simulink model "experimental_results"  (R2020b)
settings: Solver=ode1  StartTime=0.0  StopTime=60  FixedStep=0.002  RelTol=1e-3  EnableMultiTasking=on
PreLoadFcn:
  | quanser_aero_lqr
undefined symbols (not defined in the file or in its folder): HIL, qc_get_step_size
libraries: quarc_library x6
settings Model: SimulationMode=external  ExtModeTrigDuration=20000  Creator=MLevis  LastModifiedBy=ffsandva
settings SolverCC: PositivePriorityOrder=on
settings DataIOCC: LimitDataPoints=on  SaveFormat=Array  ReturnWorkspaceOutputs=off
settings OptimizationCC: LifeSpan=inf
settings DebuggingCC: SolverPrmCheckMsg=warning  SFUnexpectedBacktrackingDiag=warning  SFNoUnconditionalDefaultTransitionDiag=warning  SFExecutionAtInitializationDiag=none  ArithmeticOperatorsInVariantConditions=warning
settings HardwareCC: ProdBitPerPointer=32  ProdBitPerSizeT=32  ProdBitPerPtrDiffT=32  ProdLargestAtomicFloat=None  ProdIntDivRoundTo=Undefined  ProdEndianess=Unspecified  ProdWordSize=32  ProdHWDeviceType=32-bit Generic
settings ModelReferenceCC: PropagateSignalLabelsOutOfModel=off
settings SFSimCC: SimUseLocalCustomCode=off  CustomCodeUndefinedFunction=UseInterfaceOnly
settings RTWCC: Description=QUARC Win64 Target  SystemTargetFile=quarc_win64.tlc  TemplateMakefile=quarc_default_tmf  RTWUseLocalCustomCode=off
settings CodeAppCC: StateflowObjectComments=on
settings STFCustomTargetCC: CPPClassGenCompliant=off
settings GRTTargetCC: TargetLangStandard=C89/C90 (ANSI)  ParMdlRefBuildCompliant=off  CompOptLevelCompliant=off  CombineOutputUpdateFcns=off  MatFileLogging=off  CPPClassGenCompliant=off  GRTInterface=on  UseToolchainInfoCompliant=off  ExtMode=on  ExtModeMexFile=quarc_comm
settings ConfigComp: CovMetricSettings=dw  CovSaveCumulativeToWorkspaceVar=on  CovSaveSingleToWorkspaceVar=on  CovExternalEMLEnable=off  CovSFcnEnable=off

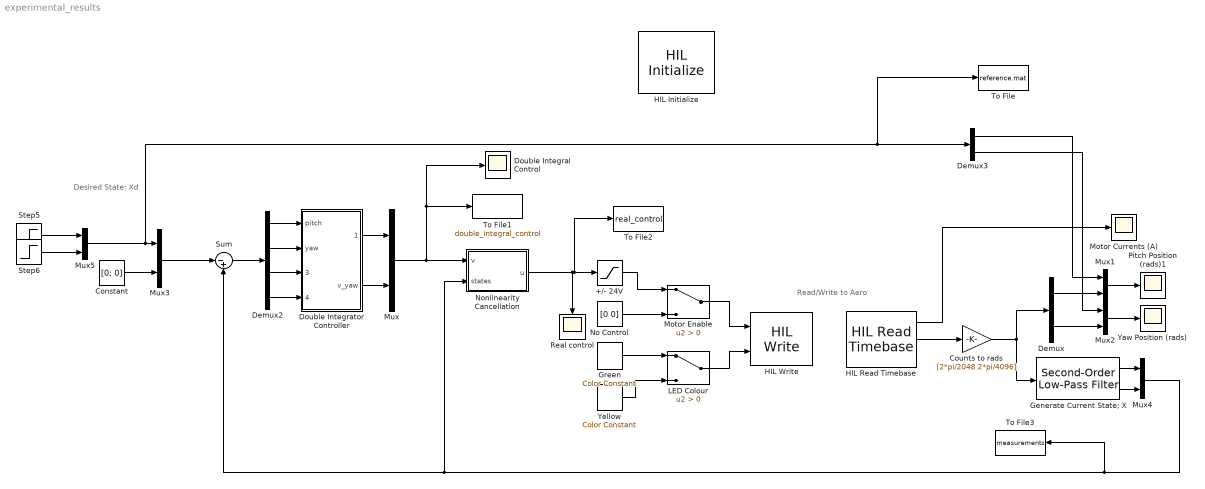
== system experimental_results ==
  note: Read/Write to Aero
  note: Desired State; Xd
  +/- 24V : Saturate  UpperLimit=24  LowerLimit=-24
  Constant : Constant  Value=[0; 0]
  Counts to rads : Gain  Gain=[2*pi/2048 2*pi/4096]
  Demux : Demux  Outputs=2
  Demux2 : Demux
  Demux3 : Demux  Outputs=2
  Double Integral Control : Scope
  Double Integrator Controller : Subsystem
  Generate Current State; X : quarc_library/Continuous/Second-Order Low-Pass Filter  params_source=Internal (dialog parameters)  input_width=50  input_zeta=0.8  input_init=0
  Green : quarc_library/Sources/Signals/Color Constant  color=[0 1 0]
      settings: SourceProductName=QUARC Targets
  HIL Initialize : quarc_library/Data Acquisition/Generic/Configuration/HIL Initialize  Priority=-99  object_name=HIL-1  board_type=quanser_aero_usb  board_number=0  board_options=""  exclusive=off  active=off  hardware_clocks=[0]  clock_modes=[]  initial_clock_frequencies=[]  set_clock_params_at_start=off  set_clock_params_at_switch_in=off  set_clock_frequencies_at_start=off  set_clock_frequencies_at_switch_in=off  analog_input_channels=[0:1]  analog_input_configurations=[]  analog_input_maximums=3  analog_input_minimums=-3  set_analog_input_params_at_start=off  set_analog_input_params_at_switch_in=off  analog_output_channels=[0:1]  analog_output_maximums=24  analog_output_minimums=-24  initial_analog_outputs=[0]  final_analog_outputs=[0]  watchdog_analog_outputs=[0]  set_analog_output_params_at_start=off  set_analog_output_params_at_switch_in=off  set_analog_outputs_at_start=on  set_analog_outputs_at_switch_in=off  set_analog_outputs_at_terminate=on  set_analog_outputs_at_switch_out=off  set_analog_outputs_on_watchdog=on  digital_input_channels=[]  digital_output_channels=[0:1]  digital_output_configuration=[]  initial_digital_outputs=[1]  final_digital_outputs=[0]  watchdog_digital_outputs=[0]  set_digital_output_params_at_start=off  set_digital_output_params_at_switch_in=off  set_digital_outputs_at_start=on  set_digital_outputs_at_switch_in=off  set_digital_outputs_at_terminate=on  set_digital_outputs_at_switch_out=off  set_digital_outputs_on_watchdog=on  encoder_channels=[0:3]  quadrature=[4]  encoder_filter_frequency=[]  initial_encoder_counts=[0]  set_encoder_params_at_start=off  set_encoder_params_at_switch_in=off  set_encoder_counts_at_start=on  set_encoder_counts_at_switch_in=off  pwm_channels=[]  pwm_modes=[]  pwm_frequency=[]  pwm_configuration=[]  pwm_alignment=[]  pwm_polarity=[]  pwm_leading_deadband=[]  pwm_trailing_deadband=[]  initial_pwm_outputs=[]  final_pwm_outputs=[]  watchdog_pwm_outputs=[]  set_pwm_params_at_start=off  set_pwm_params_at_switch_in=off  set_pwm_outputs_at_start=off  set_pwm_outputs_at_switch_in=off  set_pwm_outputs_at_terminate=off  set_pwm_outputs_at_switch_out=off  set_pwm_outputs_on_watchdog=off  other_output_channels=[11000:11002]  initial_other_outputs=[0 1 0]  final_other_outputs=[1 0 0]  watchdog_other_outputs=[0 0 1]  set_other_outputs_at_start=on  set_other_outputs_at_switch_in=off  set_other_outputs_at_terminate=on  set_other_outputs_at_switch_out=off  set_other_outputs_on_watchdog=on
  HIL Read Timebase : quarc_library/Data Acquisition/Generic/Timebases/HIL Read Timebase  object_name=HIL-1  clock=0  analog_channels=[0:1]  encoder_channels=[2:3]  digital_channels=[]  other_channels=[4000 4002 14000 14001]  active=on  vector_output=on  data_type_mode=Inherit via back propagation  encoder_data_type=double  digital_data_type=boolean  overflow_mode=Error on overflow  samples_in_buffer=max(ceil(1/qc_get_step_size), 1)
  HIL Write : quarc_library/Data Acquisition/Generic/Immediate I//O/HIL Write  object_name=HIL-1  analog_channels=[0:1]  pwm_channels=[]  digital_channels=[]  other_channels=[11000:11002]  sample_time=-1  active=off  vector_input=on
  LED Colour : Switch  Criteria=u2 > Threshold
  Motor Currents (A) : Scope
  Motor Enable : Switch  Criteria=u2 > Threshold
  Mux{,1..5} (6 alike) : Mux  Inputs=2
  No Control : Constant  Value=[0 0]
  Nonlinearity Cancellation : MATLAB Function  TreatAsAtomicUnit=on
  Pitch Position (rads)1 : Scope
  Real control : Scope
  Step5 : Step  Time=5  After=pi/6  SampleTime=0
  Step6 : Step  Time=5  After=pi/4  SampleTime=0
  Sum : Sum  Inputs=|-+
  To File : ToFile  Filename=reference.mat
  To File1 : ToFile  Filename=double_integral_control
  To File2 : ToFile  Filename=real_control
  To File3 : ToFile  Filename=measurements
  Yaw Position (rads) : Scope
  Yellow : quarc_library/Sources/Signals/Color Constant  color=[1 1 0]
      settings: SourceProductName=QUARC Targets
  wires:
  HIL Read Timebase/2 -> Counts to rads/1
  +/- 24V/1 -> Motor Enable/1
  Motor Enable/1 -> HIL Write/1
  LED Colour/1 -> HIL Write/2
  No Control/1 -> Motor Enable/3
  Green/1 -> LED Colour/1
  Yellow/1 -> LED Colour/3
  Counts to rads/1 -> Demux/1, Generate Current State; X/1
  HIL Read Timebase/1 -> Motor Currents (A)/1
  Generate Current State; X/2 -> Mux4/2
  Generate Current State; X/1 -> Mux4/1
  Demux/1 -> Mux1/2
  Mux1/1 -> Pitch Position (rads)1/1
  Demux/2 -> Mux2/2
  Mux2/1 -> Yaw Position (rads)/1
  Mux4/1 -> To File3/1, Sum/2, Nonlinearity Cancellation/2(states)
  Double Integrator Controller/1(v_pitch) -> Mux/1
  Double Integrator Controller/2(v_yaw) -> Mux/2
  Demux2/1 -> Double Integrator Controller/1(pitch)
  Demux2/2 -> Double Integrator Controller/2(yaw)
  Demux2/3 -> Double Integrator Controller/3(pitch_dot)
  Demux2/4 -> Double Integrator Controller/4(yaw_dot)
  Sum/1 -> Demux2/1
  Mux5/1 -> To File/1, Demux3/1, Mux3/1
  Constant/1 -> Mux3/2
  Mux3/1 -> Sum/1
  Demux3/1 -> Mux1/1
  Demux3/2 -> Mux2/1
  Mux/1 -> Double Integral Control/1, To File1/1, Nonlinearity Cancellation/1(v)
  Nonlinearity Cancellation/1(u) -> Real control/1, To File2/1, +/- 24V/1
  Step6/1 -> Mux5/2
  Step5/1 -> Mux5/1

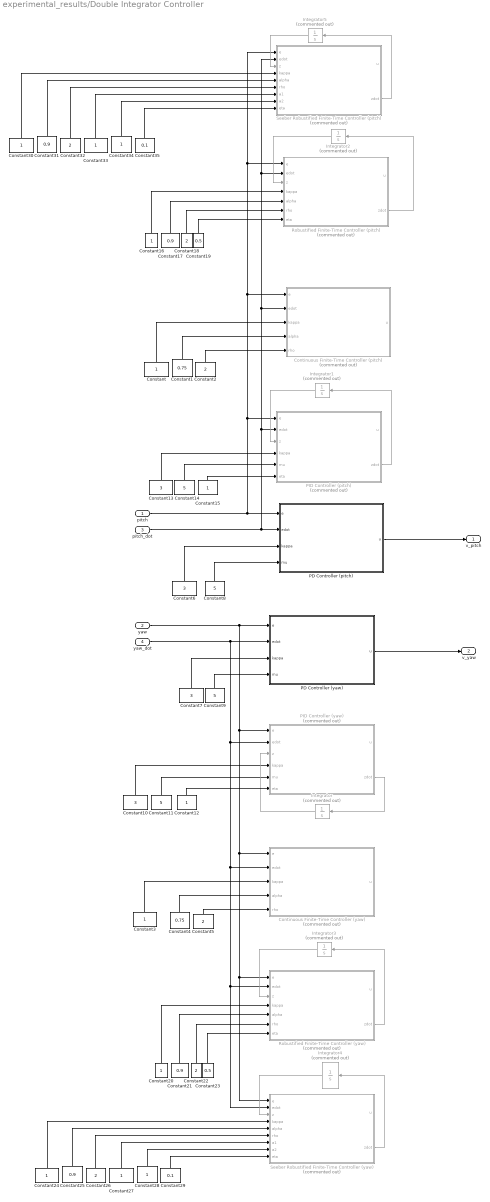
== system experimental_results/Double Integrator Controller ==
  pitch : Inport
  yaw : Inport  Port=2
  pitch_dot : Inport  Port=3
  yaw_dot : Inport  Port=4
  Constant{,3,12,15..16,20,24,27..28,30,33..34} (12 alike) : Constant
  Constant1 : Constant  Value=0.75
  Constant{6..7,10,13} (4 alike) : Constant  Value=3
  Constant{8..9,11,14} (4 alike) : Constant  Value=5
  Constant{17,21,25,31} (4 alike) : Constant  Value=0.9
  Constant{2,5,18,22,26,32} (6 alike) : Constant  Value=2
  Constant19 : Constant  Value=0.5
  Constant23 : Constant  Value=0.5
  Constant29 : Constant  Value=0.1
  Constant35 : Constant  Value=0.1
  Constant4 : Constant  Value=0.75
  Continuous Finite-Time Controller (pitch) : MATLAB Function  Commented=on  TreatAsAtomicUnit=on
  Continuous Finite-Time Controller (yaw) : MATLAB Function  Commented=on  TreatAsAtomicUnit=on
  Integrator{,1..5} (6 alike) : Integrator  Commented=on
  PD Controller (pitch) : MATLAB Function  TreatAsAtomicUnit=on
  PD Controller (yaw) : MATLAB Function  TreatAsAtomicUnit=on
  PID Controller (pitch) : MATLAB Function  Commented=on  TreatAsAtomicUnit=on
  PID Controller (yaw) : MATLAB Function  Commented=on  TreatAsAtomicUnit=on
  Robustified Finite-Time Controller (pitch) : MATLAB Function  Commented=on  TreatAsAtomicUnit=on
  Robustified Finite-Time Controller (yaw) : MATLAB Function  Commented=on  TreatAsAtomicUnit=on
  Seeber Robustified Finite-Time Controller (pitch) : MATLAB Function  Commented=on  TreatAsAtomicUnit=on
  Seeber Robustified Finite-Time Controller (yaw) : MATLAB Function  Commented=on  TreatAsAtomicUnit=on
  v_pitch : Outport
  v_yaw : Outport  Port=2
  wires:
  pitch/1 -> Seeber Robustified Finite-Time Controller (pitch)/1(e), Robustified Finite-Time Controller (pitch)/1(e), Continuous Finite-Time Controller (pitch)/1(e), PID Controller (pitch)/1(e), PD Controller (pitch)/1(e)
  Constant/1 -> Continuous Finite-Time Controller (pitch)/3(kappa)
  Constant1/1 -> Continuous Finite-Time Controller (pitch)/4(alpha)
  Constant2/1 -> Continuous Finite-Time Controller (pitch)/5(rho)
  pitch_dot/1 -> PID Controller (pitch)/2(edot), Continuous Finite-Time Controller (pitch)/2(edot), Seeber Robustified Finite-Time Controller (pitch)/2(edot), Robustified Finite-Time Controller (pitch)/2(edot), PD Controller (pitch)/2(edot)
  Constant3/1 -> Continuous Finite-Time Controller (yaw)/3(kappa)
  Constant5/1 -> Continuous Finite-Time Controller (yaw)/5(rho)
  Constant4/1 -> Continuous Finite-Time Controller (yaw)/4(alpha)
  yaw/1 -> Continuous Finite-Time Controller (yaw)/1(e), Seeber Robustified Finite-Time Controller (yaw)/1(e), Robustified Finite-Time Controller (yaw)/1(e), PID Controller (yaw)/1(e), PD Controller (yaw)/1(e)
  Constant6/1 -> PD Controller (pitch)/3(kappa)
  Constant8/1 -> PD Controller (pitch)/4(mu)
  Constant9/1 -> PD Controller (yaw)/4(mu)
  Constant7/1 -> PD Controller (yaw)/3(kappa)
  Constant10/1 -> PID Controller (yaw)/4(kappa)
  Constant11/1 -> PID Controller (yaw)/5(mu)
  PID Controller (yaw)/2(zdot) -> Integrator/1
  Integrator/1 -> PID Controller (yaw)/3(z)
  Constant12/1 -> PID Controller (yaw)/6(eta)
  yaw_dot/1 -> Continuous Finite-Time Controller (yaw)/2(edot), Robustified Finite-Time Controller (yaw)/2(edot), Seeber Robustified Finite-Time Controller (yaw)/2(edot), PID Controller (yaw)/2(edot), PD Controller (yaw)/2(edot)
  PID Controller (pitch)/2(zdot) -> Integrator1/1
  Integrator1/1 -> PID Controller (pitch)/3(z)
  Constant13/1 -> PID Controller (pitch)/4(kappa)
  Constant14/1 -> PID Controller (pitch)/5(mu)
  Constant15/1 -> PID Controller (pitch)/6(eta)
  Robustified Finite-Time Controller (pitch)/2(zdot) -> Integrator2/1
  Integrator2/1 -> Robustified Finite-Time Controller (pitch)/3(z)
  Constant16/1 -> Robustified Finite-Time Controller (pitch)/4(kappa)
  Constant17/1 -> Robustified Finite-Time Controller (pitch)/5(alpha)
  Constant18/1 -> Robustified Finite-Time Controller (pitch)/6(rho)
  Constant19/1 -> Robustified Finite-Time Controller (pitch)/7(eta)
  Constant21/1 -> Robustified Finite-Time Controller (yaw)/5(alpha)
  Robustified Finite-Time Controller (yaw)/2(zdot) -> Integrator3/1
  Constant22/1 -> Robustified Finite-Time Controller (yaw)/6(rho)
  Constant23/1 -> Robustified Finite-Time Controller (yaw)/7(eta)
  Integrator3/1 -> Robustified Finite-Time Controller (yaw)/3(z)
  Constant20/1 -> Robustified Finite-Time Controller (yaw)/4(kappa)
  Seeber Robustified Finite-Time Controller (yaw)/2(zdot) -> Integrator4/1
  Constant27/1 -> Seeber Robustified Finite-Time Controller (yaw)/7(a1)
  Constant28/1 -> Seeber Robustified Finite-Time Controller (yaw)/8(a2)
  Constant25/1 -> Seeber Robustified Finite-Time Controller (yaw)/5(alpha)
  Constant24/1 -> Seeber Robustified Finite-Time Controller (yaw)/4(kappa)
  Constant26/1 -> Seeber Robustified Finite-Time Controller (yaw)/6(rho)
  Constant29/1 -> Seeber Robustified Finite-Time Controller (yaw)/9(eta)
  Integrator4/1 -> Seeber Robustified Finite-Time Controller (yaw)/3(z)
  Seeber Robustified Finite-Time Controller (pitch)/2(zdot) -> Integrator5/1
  Constant35/1 -> Seeber Robustified Finite-Time Controller (pitch)/9(eta)
  Constant32/1 -> Seeber Robustified Finite-Time Controller (pitch)/6(rho)
  Constant30/1 -> Seeber Robustified Finite-Time Controller (pitch)/4(kappa)
  Constant31/1 -> Seeber Robustified Finite-Time Controller (pitch)/5(alpha)
  Constant33/1 -> Seeber Robustified Finite-Time Controller (pitch)/7(a1)
  Integrator5/1 -> Seeber Robustified Finite-Time Controller (pitch)/3(z)
  Constant34/1 -> Seeber Robustified Finite-Time Controller (pitch)/8(a2)
  PD Controller (pitch)/1(u) -> v_pitch/1
  PD Controller (yaw)/1(u) -> v_yaw/1

== matlab function experimental_results/Double Integrator Controller/Robustified Finite-Time Controller (yaw) ==
  data: e input; u output; edot input; z input; kappa input; alpha input; rho input; zdot output; eta input
function [u, zdot] = RobustifiedFiniteTimeController(e, edot, z, kappa, alpha, rho, eta)
    % [u, zdot] = RobustifiedFiniteTimeController(e, edot, z, kappa, alpha, rho, eta) 
    % computes the feedback control for a robustified finite-time
    % controller given the positive parameters kappa, alpha, rho and eta.
    %
    % Author:   Finn F. Sandvand
    % Date:     15th Jun 2025
    % Revisions: 

    sigma = edot + kappa * sign(e) * abs(e)^alpha;
    mu = alpha * kappa^(1/alpha) + rho;
    u = alpha * kappa^2 * sign(e) * abs(e)^(2*alpha-1) ...
        - mu * sign(sigma) * abs(sigma)^((2*alpha-1)/alpha) - eta * z;
    zdot = sign(sigma);
end

== matlab function experimental_results/Double Integrator Controller/Seeber Robustified Finite-Time Controller (yaw) ==
  data: e input; u output; edot input; z input; kappa input; alpha input; rho input; zdot output; a1 input; a2 input; eta input
function [u, zdot] = SeeberRobustifiedFiniteTimeController(e, edot, z, kappa, alpha, rho, a1, a2, eta)
    % [u, zdot] = SeeberRobustifiedFiniteTimeController(e, edot, z, kappa, alpha, rho, a1, a2, eta) 
    % computes the feedback control for a robustified finite-time
    % controller given the positive parameters kappa, alpha, rho, a1, a2
    % and eta.
    %
    % Author:   Finn F. Sandvand
    % Date:     15th Jun 2025
    % Revisions: 

    sigma = edot + kappa * sign(e) * abs(e)^alpha;
    mu = alpha * kappa^(1/alpha) + rho;
    k = alpha * kappa^2 * sign(e) * abs(e)^(2*alpha-1) ...
        - mu * sign(sigma) * abs(sigma)^((2*alpha-1)/alpha);

    h = edot / (a1 * abs(e)^(2-alpha) + a2 * abs(edot)^((2-alpha)/alpha))^((2*alpha-1)/(2-alpha));
    dhdx1 = a1 * (1-2*alpha) * abs(e)^(1-alpha) * edot / (a1 * abs(e)^(2-alpha) + a2 * abs(edot)^((2-alpha)/alpha))^((alpha+1)/(2-alpha));
    dhdx2 = 1 / (a1 * abs(e)^(2-alpha) + a2 * abs(edot)^((2-alpha)/alpha))^((2*alpha-1)/(2-alpha)) + a2 * (1-2*alpha)/alpha * sign(edot) * abs(edot)^(1/alpha) / (a1 * abs(e)^(2-alpha) + a2 * abs(edot)^((2-alpha)/alpha))^((alpha+1)/(2-alpha));

    % handle singular cases
    if isnan(dhdx1)
        dhdx1 = 0;
    end
    if isnan(dhdx2)
        dhdx2 = 0;
    end
    if isnan(h)
        h = 0;
    end

    u = k - eta * h + eta * z;
    zdot = dhdx1 * edot + dhdx2 * k;
end

== matlab function experimental_results/Double Integrator Controller/Seeber Robustified Finite-Time Controller (pitch) ==
  data: e input; u output; edot input; z input; kappa input; alpha input; rho input; zdot output; a1 input; a2 input; eta input
function [u, zdot] = SeeberRobustifiedFiniteTimeController(e, edot, z, kappa, alpha, rho, a1, a2, eta)
    % [u, zdot] = SeeberRobustifiedFiniteTimeController(e, edot, z, kappa, alpha, rho, a1, a2, eta) 
    % computes the feedback control for a robustified finite-time
    % controller given the positive parameters kappa, alpha, rho, a1, a2
    % and eta.
    %
    % Author:   Finn F. Sandvand
    % Date:     15th Jun 2025
    % Revisions: 

    sigma = edot + kappa * sign(e) * abs(e)^alpha;
    mu = alpha * kappa^(1/alpha) + rho;
    k = alpha * kappa^2 * sign(e) * abs(e)^(2*alpha-1) ...
        - mu * sign(sigma) * abs(sigma)^((2*alpha-1)/alpha);

    h = edot / (a1 * abs(e)^(2-alpha) + a2 * abs(edot)^((2-alpha)/alpha))^((2*alpha-1)/(2-alpha));
    dhdx1 = a1 * (1-2*alpha) * abs(e)^(1-alpha) * edot / (a1 * abs(e)^(2-alpha) + a2 * abs(edot)^((2-alpha)/alpha))^((alpha+1)/(2-alpha));
    dhdx2 = 1 / (a1 * abs(e)^(2-alpha) + a2 * abs(edot)^((2-alpha)/alpha))^((2*alpha-1)/(2-alpha)) + a2 * (1-2*alpha)/alpha * sign(edot) * abs(edot)^(1/alpha) / (a1 * abs(e)^(2-alpha) + a2 * abs(edot)^((2-alpha)/alpha))^((alpha+1)/(2-alpha));

    % handle singular cases
    if isnan(dhdx1)
        dhdx1 = 0;
    end
    if isnan(dhdx2)
        dhdx2 = 0;
    end
    if isnan(h)
        h = 0;
    end

    u = k - eta * h + eta * z;
    zdot = dhdx1 * edot + dhdx2 * k;
end

== matlab function experimental_results/Nonlinearity Cancellation ==
  data: v input; states input; u output
function u = NonlinearityCancellation(v, states)
    theta = states(1);
    psi = states(2);
    thetadot = states(3);
    psidot = states(4);
    
    % parameters
    g = 9.81;
    dt = 0.158;
    me = 0.2;
    dx = 0.016;
    
    ry = 0.02;
    my = 0.526;
    
    mpa = 0.146;
    lt = 0.165;
    mmt = 0.089;
    mtt = 0.089;
    mtc = 0.280;
    mrod = mmt + mtt + mtc;
    
    Ibyy = 2*mpa*dt^2 + 2*me*dt^2 + me*dx^2 + 1/12*mrod*lt^2;
    Ifyzz = 1/2*my*ry^2;
    
    M = [
        Ibyy, 0;
        0, Ifyzz + Ibyy * cos(theta)^2;
    ];
    C = [
        0, Ibyy * psidot * cos(theta)*sin(theta);
        0, -2*Ibyy * thetadot * cos(theta)*sin(theta);
    ];
    gvec = [
        dx * g * me * sin(theta);
        0;
    ];
    
    Kmtheta = 1.26e-6;
    Kttheta = 1.08e-6;
    Kmpsi = Kttheta;
    Ktpsi = Kmtheta; 

    K_omega = 17.38;
    
    B = K_omega^2 * dt * [
        Kmtheta, Kttheta;
        -Kmpsi * cos(theta), Ktpsi * cos(theta);
    ];

    d1 = 0.0031;
    d2 = 0.0075;

    D = [
        d1, 0;
        0, d2;
    ];

    q = [
        theta;
        psi;
    ];
    qdot = [
        thetadot;
        psidot;
    ];

    utilde = B \ (M*v + C * qdot + D * qdot + gvec);
    u = sign(utilde) .* sqrt(abs(utilde));
end

== matlab function experimental_results/Double Integrator Controller/Continuous Finite-Time Controller (yaw) ==
  data: e input; u output; edot input; kappa input; alpha input; rho input
function u = ContinuousFiniteTimeController(e, edot, kappa, alpha, rho)
    % u = OrbitalTerminalSlidingMode(e, edot, kappa, alpha, rho) computes
    % the feedback control for a continuous finite-time controller given 
    % the positive parameters kappa, alpha and rho.
    %
    % Author:   Finn F. Sandvand
    % Date:     15th Jun 2025
    % Revisions: 

    sigma = edot + kappa * sign(e) * abs(e)^alpha;
    mu = alpha * kappa^(1/alpha) + rho;
    u = alpha * kappa^2 * sign(e) * abs(e)^(2*alpha-1) ...
        - mu * sign(sigma) * abs(sigma)^((2*alpha-1)/alpha);
end

== matlab function experimental_results/Double Integrator Controller/PD Controller (pitch) ==
  data: e input; u output; edot input; kappa input; mu input
function u = PDController(e, edot, kappa, mu)
    % u = PDController(e, edot, kappa, mu) computes the feedback control 
    % for a Proportional-Derivative controller given the positive 
    % parameters kappa and mu.
    %
    % Author:   Finn F. Sandvand
    % Date:     15th Jun 2025
    % Revisions: 

    if kappa <= 0 || mu <= 0
        error('Error. kappa and mu must be positive');
    elseif kappa >= mu
        error('Error. kappa must be greater than mu');
    end

    sigma = edot + kappa * e;
    u = kappa^2 * e - mu * sigma;
end

== matlab function experimental_results/Double Integrator Controller/PD Controller (yaw) ==
  data: e input; u output; edot input; kappa input; mu input
function u = PDController(e, edot, kappa, mu)
    % u = PDController(e, edot, kappa, mu) computes the feedback control 
    % for a Proportional-Derivative controller given the positive 
    % parameters kappa and mu.
    %
    % Author:   Finn F. Sandvand
    % Date:     15th Jun 2025
    % Revisions: 

    if kappa <= 0 || mu <= 0
        error('Error. kappa and mu must be positive');
    elseif kappa >= mu
        error('Error. kappa must be greater than mu');
    end

    sigma = edot + kappa * e;
    u = kappa^2 * e - mu * sigma;
end

== matlab function experimental_results/Double Integrator Controller/PID Controller (yaw) ==
  data: e input; u output; edot input; z input; kappa input; mu input; eta input; zdot output
function [u, zdot] = PIDController(e, edot, z, kappa, mu, eta)
    % [u, zdot] = RobustifiedFiniteTimeController(e, edot, z, kappa, mu, eta) 
    % computes the feedback control for a Proportional-Integral-Derviative
    % controller given the positive parameters kappa, mu and eta.
    %
    % Author:   Finn F. Sandvand
    % Date:     15th Jun 2025
    % Revisions: 

    if kappa <= 0 || mu <= 0 || eta <= 0
        error('Error. kappa, mu and eta must be positive');
    elseif kappa >= mu
        error('Error. kappa must be greater than mu');
    end

    sigma = edot + kappa * e;
    u = -kappa*(mu - kappa) * e - mu * edot - eta * z;
    zdot = sigma;
end

== matlab function experimental_results/Double Integrator Controller/PID Controller (pitch) ==
  data: e input; u output; edot input; z input; kappa input; mu input; eta input; zdot output
function [u, zdot] = PIDController(e, edot, z, kappa, mu, eta)
    % [u, zdot] = RobustifiedFiniteTimeController(e, edot, z, kappa, mu, eta) 
    % computes the feedback control for a Proportional-Integral-Derviative
    % controller given the positive parameters kappa, mu and eta.
    %
    % Author:   Finn F. Sandvand
    % Date:     15th Jun 2025
    % Revisions: 

    if kappa <= 0 || mu <= 0 || eta <= 0
        error('Error. kappa, mu and eta must be positive');
    elseif kappa >= mu
        error('Error. kappa must be greater than mu');
    end

    sigma = edot + kappa * e;
    u = -kappa*(mu - kappa) * e - mu * edot - eta * z;
    zdot = sigma;
end

== matlab function experimental_results/Double Integrator Controller/Continuous Finite-Time Controller (pitch) ==
  data: e input; u output; edot input; kappa input; alpha input; rho input
function u = ContinuousFiniteTimeController(e, edot, kappa, alpha, rho)
    % u = OrbitalTerminalSlidingMode(e, edot, kappa, alpha, rho) computes
    % the feedback control for a continuous finite-time controller given 
    % the positive parameters kappa, alpha and rho.
    %
    % Author:   Finn F. Sandvand
    % Date:     15th Jun 2025
    % Revisions: 

    sigma = edot + kappa * sign(e) * abs(e)^alpha;
    mu = alpha * kappa^(1/alpha) + rho;
    u = alpha * kappa^2 * sign(e) * abs(e)^(2*alpha-1) ...
        - mu * sign(sigma) * abs(sigma)^((2*alpha-1)/alpha);
end

== matlab function experimental_results/Double Integrator Controller/Robustified Finite-Time Controller (pitch) ==
  data: e input; u output; edot input; z input; kappa input; alpha input; rho input; zdot output; eta input
function [u, zdot] = RobustifiedFiniteTimeController(e, edot, z, kappa, alpha, rho, eta)
    % [u, zdot] = RobustifiedFiniteTimeController(e, edot, z, kappa, alpha, rho, eta) 
    % computes the feedback control for a robustified finite-time
    % controller given the positive parameters kappa, alpha, rho and eta.
    %
    % Author:   Finn F. Sandvand
    % Date:     15th Jun 2025
    % Revisions: 

    sigma = edot + kappa * sign(e) * abs(e)^alpha;
    mu = alpha * kappa^(1/alpha) + rho;
    u = alpha * kappa^2 * sign(e) * abs(e)^(2*alpha-1) ...
        - mu * sign(sigma) * abs(sigma)^((2*alpha-1)/alpha) - eta * z;
    zdot = sign(sigma);
end
